simulink model "Unicycle_b"  (Simulink 8.9)
settings: Solver=VariableStepAuto  StartTime=0.0  StopTime=T  RelTol=1e-3
values from neighbouring files (symbols this model uses):
  theta0 = theta(end)    [Simulation.m]    (also in TestSimulink.m)
  x0 = x(end)    [Simulation.m]    (also in TestSimulink.m)
  y0 = y(end)    [Simulation.m]    (also in TestSimulink.m)
settings Model: SuppressorTable=22 serialization::archive 11 0 6 0 0 0 0 0  Creator=Bruno Alves  LastModifiedBy=joaogarcia
settings DataIOCC: LimitDataPoints=off  SaveFormat=Dataset  SignalLoggingSaveFormat=Dataset
settings OptimizationCC: LifeSpan=auto
settings DebuggingCC: UnderspecifiedInitializationDetection=Simplified  MergeDetectMultiDrivingBlocksExec=error  FcnCallInpInsideContextMsg=error  StateNameClashWarn=none  SFUnexpectedBacktrackingDiag=error  SFNoUnconditionalDefaultTransitionDiag=error  SFExecutionAtInitializationDiag=warning
settings HardwareCC: ProdBitPerPointer=64  ProdBitPerSizeT=64  ProdBitPerPtrDiffT=64  ProdLargestAtomicFloat=Float  ProdIntDivRoundTo=Zero  ProdEndianess=LittleEndian  ProdWordSize=64  ProdHWDeviceType=Intel->x86-64 (Windows64)
settings ModelReferenceCC: PropagateSignalLabelsOutOfModel=on
settings GRTTargetCC: TargetLangStandard=C99 (ISO)  GeneratePreprocessorConditionals=Use local settings  CombineOutputUpdateFcns=on  GRTInterface=off
settings ConfigComp: CovMetricSettings=dwe  CovHtmlReporting=off  CovSaveCumulativeToWorkspaceVar=off  CovSaveSingleToWorkspaceVar=off  CovExternalEMLEnable=on

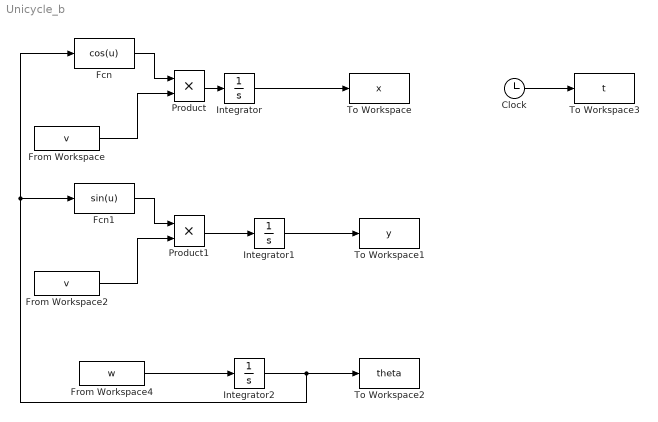
== system Unicycle_b ==
  Clock : Clock
  Fcn : Fcn  Expr=cos(u)
  Fcn1 : Fcn  Expr=sin(u)
  From Workspace : FromWorkspace  VariableName=v  SampleTime=0
  From Workspace2 : FromWorkspace  VariableName=v  SampleTime=0
  From Workspace4 : FromWorkspace  VariableName=w  SampleTime=0
  Integrator : Integrator  InitialCondition=x0
  Integrator1 : Integrator  InitialCondition=y0
  Integrator2 : Integrator  InitialCondition=theta0
  Product : Product
  Product1 : Product
  To Workspace : ToWorkspace  VariableName=x  SampleTime=-1
  To Workspace1 : ToWorkspace  VariableName=y  SampleTime=-1
  To Workspace2 : ToWorkspace  VariableName=theta  SampleTime=-1
  To Workspace3 : ToWorkspace  VariableName=t  SampleTime=-1
  wires:
  Product/1 -> Integrator/1
  Fcn/1 -> Product/1
  From Workspace/1 -> Product/2
  Integrator/1 -> To Workspace/1
  Product1/1 -> Integrator1/1
  From Workspace2/1 -> Product1/2
  Fcn1/1 -> Product1/1
  Integrator1/1 -> To Workspace1/1
  Integrator2/1 -> Fcn/1, Fcn1/1, To Workspace2/1
  From Workspace4/1 -> Integrator2/1
  Clock/1 -> To Workspace3/1
